simulink model "Ejercicio16_20_02_17"  (R2013a)
settings: Solver=ode45  StartTime=0.0  StopTime=10.0  RelTol=1e-3
settings Model: Creator=Miguel  LastModifiedBy=Miguel

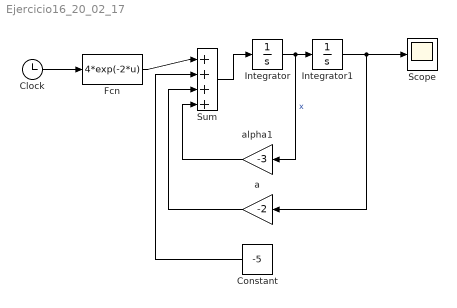
== system Ejercicio16_20_02_17 ==
  Clock : Clock
  Constant : Constant  Value=-5
  Fcn : Fcn  Expr=4*exp(-2*u)
  Integrator : Integrator  InitialCondition=-1
  Integrator1 : Integrator  InitialCondition=2
  Scope : Scope
      settings: ShowLegends=on  TimeRange=10
  Sum : Sum  Inputs=|++++
  a : Gain  Gain=-2
  alpha1 : Gain  Gain=-3
  wires:
  Sum/1 -> Integrator/1
  Integrator/1 -> alpha1/1, Integrator1/1  "x"
  Integrator1/1 -> a/1, Scope/1
  Fcn/1 -> Sum/1
  alpha1/1 -> Sum/4
  a/1 -> Sum/3
  Constant/1 -> Sum/2
  Clock/1 -> Fcn/1
